simulink model "DancingRobots"  (R2013b)
settings: Solver=ode45  StartTime=0.0  StopTime=10.0  RelTol=1e-3
settings Model: Creator=Justyna  LastModifiedBy=Justyna
settings DebuggingCC: StateNameClashWarn=warning

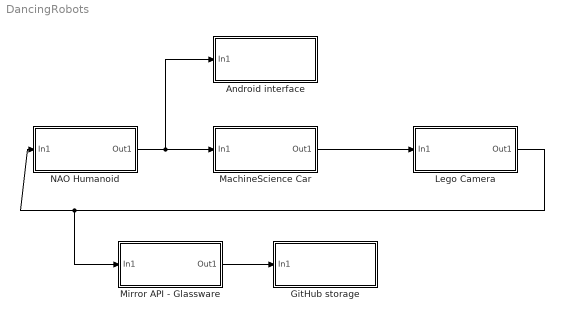
== system DancingRobots ==
  Android interface : Subsystem
  GitHub storage : Subsystem
  "Lego Camera " : Subsystem
  MachineScience Car : Subsystem
  Mirror API - Glassware : Subsystem
  NAO Humanoid : Subsystem
  wires:
  NAO Humanoid/1(Out1) -> Android interface/1(In1), MachineScience Car/1(In1)
  MachineScience Car/1(Out1) -> "Lego Camera "/1(In1)
  "Lego Camera "/1(Out1) -> Mirror API - Glassware/1(In1), NAO Humanoid/1(In1)
  Mirror API - Glassware/1(Out1) -> GitHub storage/1(In1)

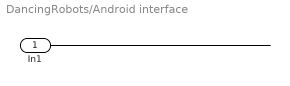
== system DancingRobots/Android interface ==
  In1 : Inport
  wires:
  In1/1 -> ?

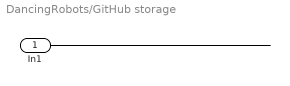
== system DancingRobots/GitHub storage ==
  In1 : Inport
  wires:
  In1/1 -> ?

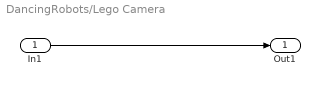
== system DancingRobots/Lego Camera  ==
  In1 : Inport
  Out1 : Outport
  wires:
  In1/1 -> Out1/1

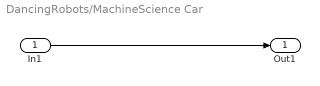
== system DancingRobots/MachineScience Car ==
  In1 : Inport
  Out1 : Outport
  wires:
  In1/1 -> Out1/1

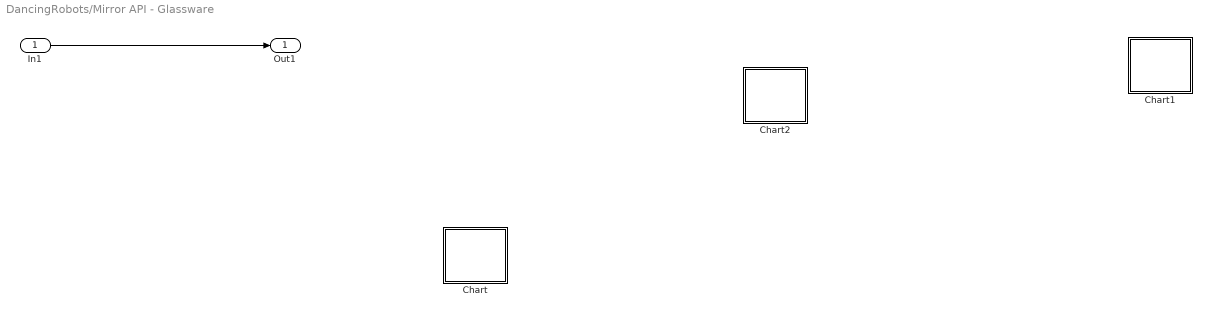
== system DancingRobots/Mirror API - Glassware ==
  In1 : Inport
  Chart : Stateflow chart  TreatAsAtomicUnit=on
  Chart1 : Stateflow chart  TreatAsAtomicUnit=on
  Chart2 : Stateflow chart  TreatAsAtomicUnit=on
  Out1 : Outport
  wires:
  In1/1 -> Out1/1

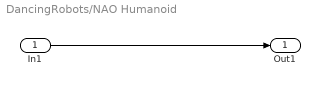
== system DancingRobots/NAO Humanoid ==
  In1 : Inport
  Out1 : Outport
  wires:
  In1/1 -> Out1/1

== stateflow chart DancingRobots/Mirror API - Glassware/Chart ==
  state start
    engine
  state drive
    forwards
  state drive
    backwards
  state stop
  state stop
    engine
  (default) -> start
  start -> stop [order 2]
  stop -> start
  start -> drive [order 3]
  start -> drive [order 1]
  drive -> stop
  stop -> drive [order 2]
  drive -> stop
  stop -> drive [order 1]
  stop -> stop [order 3]

== stateflow chart DancingRobots/Mirror API - Glassware/Chart1 ==

== stateflow chart DancingRobots/Mirror API - Glassware/Chart2 ==
